simulink model "rlVarth_siml"  (R2020b)
settings: Solver=ode23t  StartTime=0.0  StopTime=Tf  RelTol=1e-2
model workspace: external: MAT-File C:\PhD\Variable Threshold\demo_rl.mat (data not in the file)
values from neighbouring files (symbols this model uses):
  A = [1.0000    0.1000;0    1.0000]    [RLenv.m]    (also in RlEnvModel.m; system.mat = [0.6278  -0.0259; 0.4644  0.7071]; systems_with_noise.m = [1.0000    0.1000; 0    1.0000])
  actorAtk = rlDeterministicActorRepresentation(actorNetwork,obsInfo{1,1},actInfo{1,1},'Observation',{'State'},'Action',{'Action'},actorOptions)    [demo_rl.m]    (also in main_rl.m = rlDeterministicActorRepresentation(actorNetwork,obsInfo{1,1}; main_rl_func_modified.m = rlDeterministicActorRepresentation(actorNetwork,obsInfo{1,1}; new_main_rl.m = rlDeterministicActorRepresentation(actorNetwork,obsInfo{1,1})
  actorCon = rlDeterministicActorRepresentation(actorNetwork,obsInfo{1,2},actInfo{1,2},'Observation',{'State'},'Action',{'Action'},actorOptions)    [demo_rl.m]    (also in main_rl.m = rlDeterministicActorRepresentation(actorNetwork,obsInfo{1,2}; main_rl_func_modified.m = rlDeterministicActorRepresentation(actorNetwork,obsInfo{1,2}; new_main_rl.m = rlDeterministicActorRepresentation(actorNetwork,obsInfo{1,2})
  actorDtc = rlDeterministicActorRepresentation(actorNetwork,obsInfo{1,3},actInfo{1,3},'Observation',{'State'},'Action',{'Action'},actorOptions)    [demo_rl.m]    (also in main_rl.m = rlDeterministicActorRepresentation(actorNetwork,obsInfo{1,3}; main_rl_func_modified.m = rlDeterministicActorRepresentation(actorNetwork,obsInfo{1,3}; new_main_rl.m = rlDeterministicActorRepresentation(actorNetwork,obsInfo{1,3})
  actuatorRange = [36]    [RLenv.m]    (also in RlEnvModel.m; system.mat = [0.8125 10000])
  agentOpts = rlDDPGAgentOptions(     'SampleTime',Ts,     'TargetSmoothFactor',1e-3,     'DiscountFactor',1.0,      'MiniBatchSize',64,      'ExperienceBufferLength',1e6)    [demo_rl.m]    (also in main_rl.m = rlDDPGAgentOptions(     'SampleTime',Ts,     'TargetSmoothFa; main_rl_func_modified.m = rlDDPGAgentOptions(     'SampleTime',Ts,     'TargetSmoothFa; new_main_rl.m = rlDDPGAgentOptions(     'SampleTime',Ts,     'TargetSmoothFa)
  B = [0.0050;0.1000]    [RLenv.m]    (also in RlEnvModel.m; system.mat = [0.1246  -2.8e-07; 3.2763  1.6e-05]; systems_with_noise.m = [0.0050; 0.1000])
  C = [1 0]    [RLenv.m]    (also in RlEnvModel.m; system.mat = [0  1; -338.7813  1.1293]; systems_with_noise.m)
  criticAtk = rlQValueRepresentation(criticNetwork,obsInfo{1,1},actInfo{1,1},'Observation',{'State'},'Action',{'Action'},criticOpts)    [demo_rl.m]    (also in main_rl.m = rlQValueRepresentation(criticNetwork,obsInfo{1,1},actInfo{1,; main_rl_func_modified.m = rlQValueRepresentation(criticNetwork,obsInfo{1,1},actInfo{1,; new_main_rl.m = rlQValueRepresentation(criticNetwork,obsInfo{1,1},actInfo{1,)
  criticCon = rlQValueRepresentation(criticNetwork,obsInfo{1,2},actInfo{1,2},'Observation',{'State'},'Action',{'Action'},criticOpts)    [demo_rl.m]    (also in main_rl.m = rlQValueRepresentation(criticNetwork,obsInfo{1,2},actInfo{1,; main_rl_func_modified.m = rlQValueRepresentation(criticNetwork,obsInfo{1,2},actInfo{1,; new_main_rl.m = rlQValueRepresentation(criticNetwork,obsInfo{1,2},actInfo{1,)
  criticDtc = rlQValueRepresentation(criticNetwork,obsInfo{1,3},actInfo{1,3},'Observation',{'State'},'Action',{'Action'},criticOpts)    [demo_rl.m]    (also in main_rl.m = rlQValueRepresentation(criticNetwork,obsInfo{1,3},actInfo{1,; main_rl_func_modified.m = rlQValueRepresentation(criticNetwork,obsInfo{1,3},actInfo{1,; new_main_rl.m = rlQValueRepresentation(criticNetwork,obsInfo{1,3},actInfo{1,)
  D = [0]    [RLenv.m]    (also in RlEnvModel.m; system.mat = [0  0; 169.3907  0]; systems_with_noise.m)
  K = [16.0302    5.6622]    [RLenv.m]    (also in RlEnvModel.m; system.mat = [5.261  -0.023; -414911.26  57009.48]; systems_with_noise.m)
  L = [0.9902;0.9892]    [RLenv.m]    (also in RlEnvModel.m; system.mat = [-2.708e-11  -6.3612e-10; 3.3671e-10  5.56308e-09]; systems_with_noise.m = [0.9902; 0.9892])
  sensorRange = [30000]    [RLenv.m]    (also in RlEnvModel.m; system.mat = [2.5 15])
  Ts = 0.1    [RLenv.m]    (also in RlEnvModel.m; demo_rl.m; main_rl.m = s.Ts; main_rl_func_modified.m = s.Ts)
undefined symbols (not defined in the file or in its folder): esp_env, rlDDPGAgent
libraries: rllib x3, simulink x2
settings Model: Creator=The MathWorks, Inc.  LastModifiedBy=IIT_KGP_CSE_FM_LAB

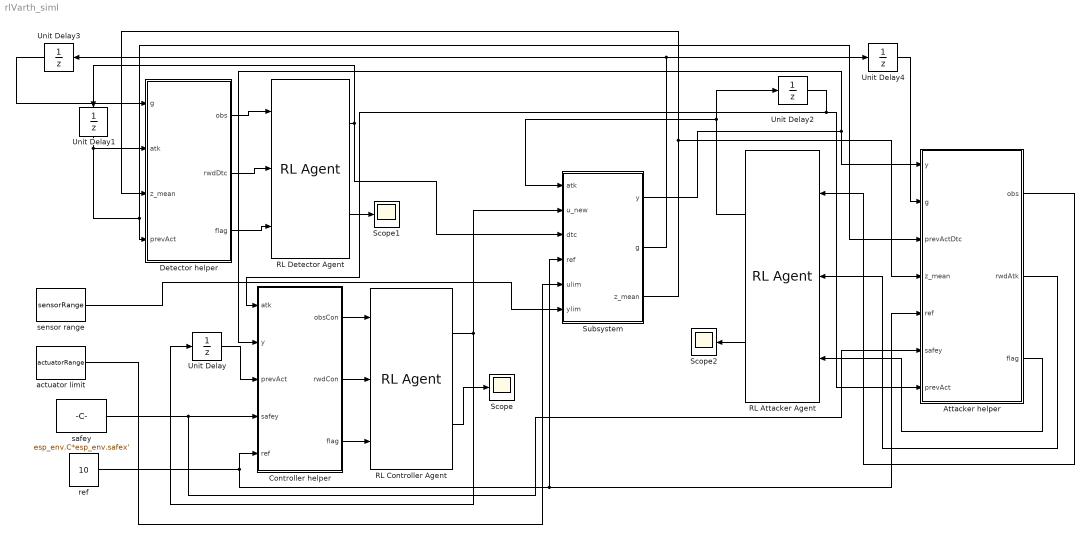
== system rlVarth_siml ==
  Attacker helper : Subsystem
  Controller helper : Subsystem
  Detector helper : Subsystem
  RL Attacker Agent : rllib/RL Agent  Agent=rlDDPGAgent(actorAtk,criticAtk,agentOpts)  ProvideReward=on  ProvideIsDone=on  ProvideCumRwd=on  TreatAsDirectFeedthrough=on  CollectLoggedSignals=on  CollectModelStates=on
  RL Controller Agent : rllib/RL Agent  Agent=rlDDPGAgent(actorCon,criticCon,agentOpts)  ProvideReward=on  ProvideIsDone=on  ProvideCumRwd=on  TreatAsDirectFeedthrough=on  CollectLoggedSignals=on  CollectModelStates=on
  RL Detector Agent : rllib/RL Agent  Agent=rlDDPGAgent(actorDtc,criticDtc,agentOpts)  ProvideReward=on  ProvideIsDone=on  ProvideCumRwd=on  TreatAsDirectFeedthrough=on  CollectLoggedSignals=on  CollectModelStates=on
  Scope : Scope
  Scope1 : Scope
  Scope2 : Scope
  Subsystem : Subsystem
  Unit Delay{,1..4} (5 alike) : UnitDelay  SampleTime=-1  HasFrameUpgradeWarning=on
  actuator limit : Constant  Value=actuatorRange
  ref : Constant  Value=10
  safey : Constant  Value=esp_env.C*esp_env.safex'
  sensor range : Constant  Value=sensorRange
  wires:
  RL Attacker Agent/1 -> Subsystem/1(atk), Unit Delay2/1
  ref/1 -> Attacker helper/5(ref), Subsystem/4(ref), Controller helper/5(ref)
  RL Controller Agent/1 -> Subsystem/2(u_new), Unit Delay/1
  RL Detector Agent/1 -> Subsystem/3(dtc), Unit Delay1/1
  RL Controller Agent/2 -> Scope/1
  RL Detector Agent/2 -> Scope1/1
  RL Attacker Agent/2 -> Scope2/1
  Unit Delay1/1 -> Attacker helper/3(prevActDtc), Detector helper/4(prevAct), Detector helper/2(atk)
  safey/1 -> Attacker helper/6(safey), Controller helper/4(safey)
  Subsystem/1(y) -> Attacker helper/1(y), Controller helper/2(y)
  Subsystem/2(g) -> Unit Delay4/1, Unit Delay3/1
  Subsystem/3(z_mean) -> Attacker helper/4(z_mean), Detector helper/3(z_mean)
  Detector helper/1(obs) -> RL Detector Agent/1
  Detector helper/2(rwdDtc) -> RL Detector Agent/2
  Detector helper/3(flag) -> RL Detector Agent/3
  Unit Delay2/1 -> Attacker helper/7(prevAct), Controller helper/1(atk)
  Unit Delay/1 -> Controller helper/3(prevAct)
  Controller helper/1(obsCon) -> RL Controller Agent/1
  Controller helper/2(rwdCon) -> RL Controller Agent/2
  Controller helper/3(flag) -> RL Controller Agent/3
  Attacker helper/1(obs) -> RL Attacker Agent/1
  Attacker helper/2(rwdAtk) -> RL Attacker Agent/2
  Attacker helper/3(flag) -> RL Attacker Agent/3
  Unit Delay3/1 -> Detector helper/1(g)
  Unit Delay4/1 -> Attacker helper/2(g)
  sensor range/1 -> Subsystem/6(ylim)
  actuator limit/1 -> Subsystem/5(ulim)

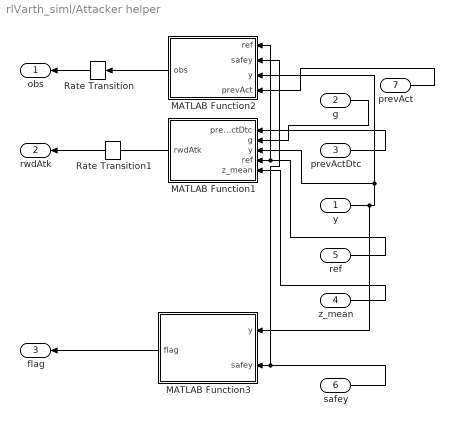
== system rlVarth_siml/Attacker helper ==
  y : Inport
  g : Inport  Port=2
  prevActDtc : Inport  Port=3
  z_mean : Inport  Port=4
  ref : Inport  Port=5
  safey : Inport  Port=6
  prevAct : Inport  Port=7
  MATLAB Function1 : MATLAB Function  TreatAsAtomicUnit=on
  MATLAB Function2 : MATLAB Function  TreatAsAtomicUnit=on
  MATLAB Function3 : MATLAB Function  TreatAsAtomicUnit=on
  Rate Transition : RateTransition
  Rate Transition1 : RateTransition
  obs : Outport
  rwdAtk : Outport  Port=2
  flag : Outport  Port=3
  wires:
  y/1 -> MATLAB Function2/3(y), MATLAB Function1/3(y), MATLAB Function3/1(y)
  g/1 -> MATLAB Function1/2(g)
  ref/1 -> MATLAB Function2/1(ref), MATLAB Function1/4(ref)
  MATLAB Function1/1(rwdAtk) -> rwdAtk/1
  z_mean/1 -> MATLAB Function1/5(z_mean)
  MATLAB Function3/1(flag) -> flag/1
  MATLAB Function2/1(obs) -> Rate Transition/1
  prevActDtc/1 -> MATLAB Function1/1(prevActDtc)
  safey/1 -> MATLAB Function2/2(safey), MATLAB Function3/2(safey)
  prevAct/1 -> MATLAB Function2/4(prevAct)
  Rate Transition/1 -> obs/1

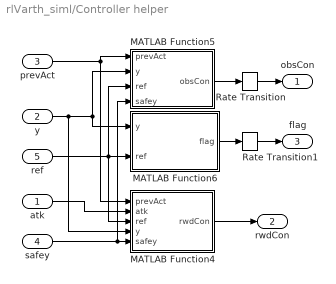
== system rlVarth_siml/Controller helper ==
  atk : Inport
  y : Inport  Port=2
  prevAct : Inport  Port=3
  safey : Inport  Port=4
  ref : Inport  Port=5
  MATLAB Function4 : MATLAB Function  TreatAsAtomicUnit=on
  MATLAB Function5 : MATLAB Function  TreatAsAtomicUnit=on
  MATLAB Function6 : MATLAB Function  TreatAsAtomicUnit=on
  Rate Transition : RateTransition
  Rate Transition1 : RateTransition
  obsCon : Outport
  rwdCon : Outport  Port=2
  flag : Outport  Port=3
  wires:
  ref/1 -> MATLAB Function4/3(ref), MATLAB Function6/2(ref), MATLAB Function5/3(ref)
  safey/1 -> MATLAB Function5/4(safey), MATLAB Function4/5(safey)
  MATLAB Function6/1(flag) -> Rate Transition1/1
  MATLAB Function4/1(rwdCon) -> rwdCon/1
  MATLAB Function5/1(obsCon) -> Rate Transition/1
  y/1 -> MATLAB Function6/1(y), MATLAB Function5/2(y), MATLAB Function4/4(y)
  prevAct/1 -> MATLAB Function4/1(prevAct), MATLAB Function5/1(prevAct)
  atk/1 -> MATLAB Function4/2(atk)
  Rate Transition/1 -> obsCon/1
  Rate Transition1/1 -> flag/1

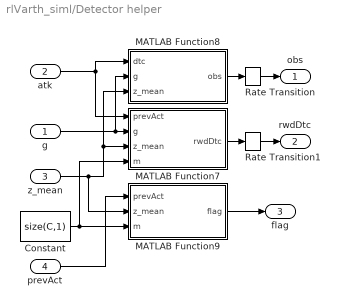
== system rlVarth_siml/Detector helper ==
  g : Inport
  atk : Inport  Port=2
  z_mean : Inport  Port=3
  prevAct : Inport  Port=4
  Constant : Constant  Value=size(C,1)  SampleTime=Ts
  MATLAB Function7 : MATLAB Function  TreatAsAtomicUnit=on
  MATLAB Function8 : MATLAB Function  TreatAsAtomicUnit=on
  MATLAB Function9 : MATLAB Function  TreatAsAtomicUnit=on
  Rate Transition : RateTransition  OutPortSampleTime=Ts
  Rate Transition1 : RateTransition
  obs : Outport
  rwdDtc : Outport  Port=2
  flag : Outport  Port=3
  wires:
  atk/1 -> MATLAB Function8/1(dtc), MATLAB Function7/1(prevAct)
  Constant/1 -> MATLAB Function9/3(m), MATLAB Function7/4(m)
  prevAct/1 -> MATLAB Function9/1(prevAct)
  z_mean/1 -> MATLAB Function9/2(z_mean), MATLAB Function7/3(z_mean), MATLAB Function8/3(z_mean)
  MATLAB Function8/1(obs) -> Rate Transition/1
  MATLAB Function7/1(rwdDtc) -> Rate Transition1/1
  g/1 -> MATLAB Function8/2(g), MATLAB Function7/2(g)
  MATLAB Function9/1(flag) -> flag/1
  Rate Transition/1 -> obs/1
  Rate Transition1/1 -> rwdDtc/1

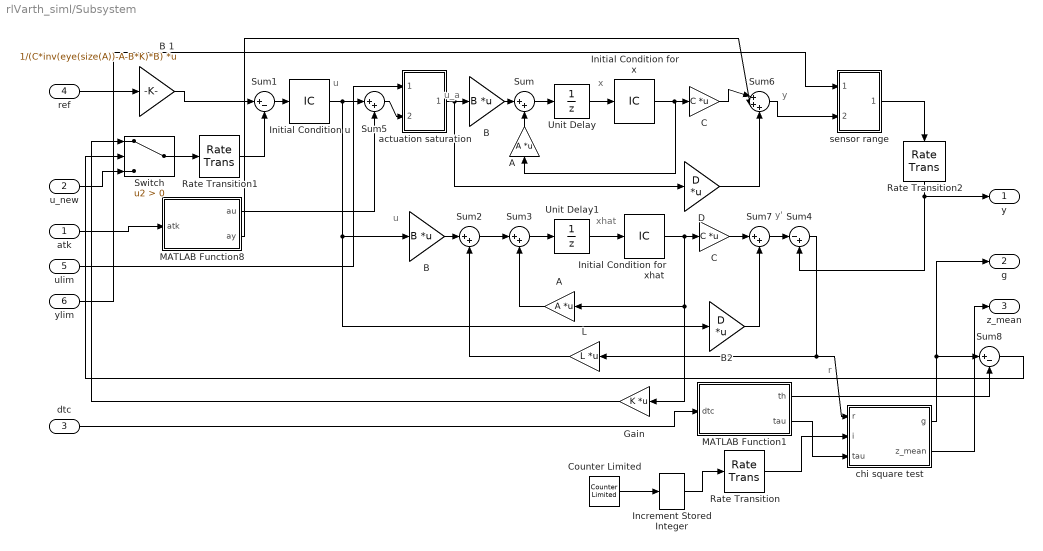
== system rlVarth_siml/Subsystem ==
  note: y
  note: r
  note: y'
  note: u
  note: u
  note: x
  note: xhat
  note: u_a
  atk : Inport
  u_new : Inport  Port=2
  dtc : Inport  Port=3
  ref : Inport  Port=4
  ulim : Inport  Port=5
  ylim : Inport  Port=6
  A : Gain  Gain=A  Multiplication=Matrix(K*u)
  "A " : Gain  Gain=A  Multiplication=Matrix(K*u)
  B : Gain  Gain=B  Multiplication=Matrix(K*u)
  "B " : Gain  Gain=B  Multiplication=Matrix(K*u)
  B 1 : Gain  Gain=1/(C*inv(eye(size(A))-A-B*K)*B)  Multiplication=Matrix(K*u)
  B2 : Gain  Gain=D  Multiplication=Matrix(K*u)
  C : Gain  Gain=C  Multiplication=Matrix(K*u)
  "C " : Gain  Gain=C  Multiplication=Matrix(K*u)
  Counter Limited : simulink/Sources/Counter Limited  uplimit=1/Ts-1  tsamp=Ts
  D : Gain  Gain=D  Multiplication=Matrix(K*u)
  Gain : Gain  Gain=K  Multiplication=Matrix(K*u)
  Increment Stored Integer : simulink/Additional Math & Discrete/Additional Math: Increment - Decrement/Increment Stored Integer
  Initial Condition u : InitialCondition  Value=zeros(size(B,2),1)
  Initial Condition for x : InitialCondition  Value=[0;0]
  Initial Condition for xhat : InitialCondition  Value=[0;0]
  L : Gain  Gain=L  Multiplication=Matrix(K*u)
  MATLAB Function1 : MATLAB Function  TreatAsAtomicUnit=on
  MATLAB Function8 : MATLAB Function  TreatAsAtomicUnit=on
  Rate Transition : RateTransition  OutPortSampleTime=Ts
  Rate Transition1 : RateTransition  OutPortSampleTime=Ts
  Rate Transition2 : RateTransition  OutPortSampleTime=Ts
  Sum{,2..3,5,7} (5 alike) : Sum  Inputs=|++
  Sum1 : Sum  Inputs=|+-
  Sum4 : Sum  Inputs=|-+
  Sum6 : Sum  Inputs=|+++
  Sum8 : Sum  Inputs=|+-
  Switch : Switch  Criteria=u2 > Threshold
  Unit Delay : UnitDelay  SampleTime=-1  HasFrameUpgradeWarning=on
  Unit Delay1 : UnitDelay  SampleTime=-1  HasFrameUpgradeWarning=on
  actuation saturation : Subsystem
  chi square test : Subsystem
  sensor range : Subsystem
  y : Outport
  g : Outport  Port=2
  z_mean : Outport  Port=3
  wires:
  Initial Condition for xhat/1 -> C/1, A/1, Gain/1
  L/1 -> Sum2/2
  "C "/1 -> Sum6/1
  D/1 -> Sum6/3
  u_new/1 -> Switch/3
  Unit Delay1/1 -> Initial Condition for xhat/1
  Sum7/1 -> Sum4/1
  Sum4/1 -> chi square test/1(r), L/1
  Sum3/1 -> Unit Delay1/1
  Unit Delay/1 -> Initial Condition for x/1
  Sum2/1 -> Sum3/1
  Sum1/1 -> Initial Condition u/1
  Initial Condition u/1 -> B/1, B2/1, Sum5/1
  Gain/1 -> Switch/1
  B2/1 -> Sum7/2
  actuation saturation/1(Out1) -> D/1, "B "/1
  A/1 -> Sum3/2
  Sum5/1 -> actuation saturation/2(In3)
  "B "/1 -> Sum/1
  Sum6/1 -> sensor range/2(In3)
  C/1 -> Sum7/1
  "A "/1 -> Sum/2
  Initial Condition for x/1 -> "C "/1, "A "/1
  ref/1 -> B 1/1
  B/1 -> Sum2/1
  Switch/1 -> Rate Transition1/1
  Sum/1 -> Unit Delay/1
  Sum8/1 -> Switch/2
  atk/1 -> MATLAB Function8/1(atk)
  MATLAB Function8/1(au) -> Sum5/2
  MATLAB Function8/2(ay) -> Sum6/2
  B 1/1 -> Sum1/1
  dtc/1 -> MATLAB Function1/1(dtc)
  MATLAB Function1/2(tau) -> chi square test/3(tau)
  chi square test/1(g) -> g/1, Sum8/1
  MATLAB Function1/1(th) -> Sum8/2
  ulim/1 -> actuation saturation/1(lim)
  sensor range/1(y_obs) -> Rate Transition2/1
  ylim/1 -> sensor range/1(lim)
  chi square test/2(z_mean) -> z_mean/1
  Increment Stored Integer/1 -> Rate Transition/1
  Counter Limited/1 -> Increment Stored Integer/1
  Rate Transition/1 -> chi square test/2(i)
  Rate Transition1/1 -> Sum1/2
  Rate Transition2/1 -> y/1, Sum4/2

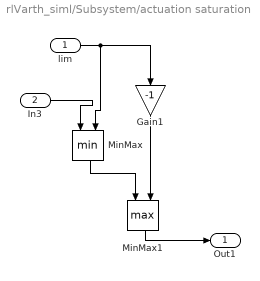
== system rlVarth_siml/Subsystem/actuation saturation ==
  lim : Inport
  In3 : Inport  Port=2
  Gain1 : Gain  Gain=-1
  MinMax : MinMax  Inputs=2
  MinMax1 : MinMax  Function=max  Inputs=2
  Out1 : Outport
  wires:
  Gain1/1 -> MinMax1/2
  MinMax/1 -> MinMax1/1
  MinMax1/1 -> Out1/1
  lim/1 -> Gain1/1, MinMax/2
  In3/1 -> MinMax/1

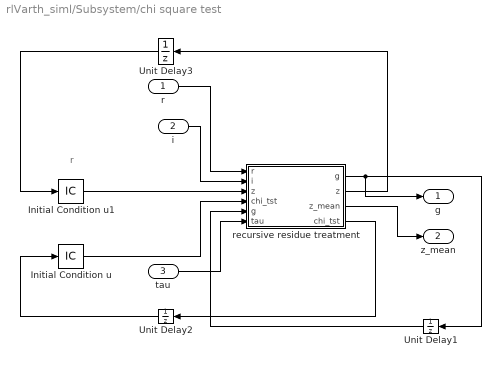
== system rlVarth_siml/Subsystem/chi square test ==
  note: r
  r : Inport
  i : Inport  Port=2
  tau : Inport  Port=3
  Initial Condition u : InitialCondition  Value=[0]
  Initial Condition u1 : InitialCondition  Value=[0]
  Unit Delay1 : UnitDelay  SampleTime=Ts  HasFrameUpgradeWarning=on
  Unit Delay2 : UnitDelay  SampleTime=Ts  HasFrameUpgradeWarning=on
  Unit Delay3 : UnitDelay  InitialCondition=[0]  SampleTime=Ts  HasFrameUpgradeWarning=on
  recursive residue treatment : MATLAB Function  TreatAsAtomicUnit=on
  g : Outport
  z_mean : Outport  Port=2
  wires:
  Unit Delay2/1 -> Initial Condition u/1
  Initial Condition u1/1 -> recursive residue treatment/3("z ")
  r/1 -> recursive residue treatment/1(r)
  Unit Delay1/1 -> recursive residue treatment/5("g ")
  Initial Condition u/1 -> recursive residue treatment/4("chi_tst ")
  Unit Delay3/1 -> Initial Condition u1/1
  recursive residue treatment/3(z_mean) -> z_mean/1
  i/1 -> recursive residue treatment/2(i)
  recursive residue treatment/4(chi_tst) -> Unit Delay2/1
  tau/1 -> recursive residue treatment/6(tau)
  recursive residue treatment/2(z) -> Unit Delay3/1
  recursive residue treatment/1(g) -> Unit Delay1/1, g/1

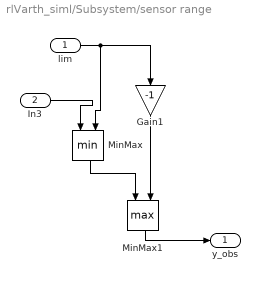
== system rlVarth_siml/Subsystem/sensor range ==
  lim : Inport
  In3 : Inport  Port=2
  Gain1 : Gain  Gain=-1
  MinMax : MinMax  Inputs=2
  MinMax1 : MinMax  Function=max  Inputs=2
  y_obs : Outport
  wires:
  Gain1/1 -> MinMax1/2
  MinMax/1 -> MinMax1/1
  MinMax1/1 -> y_obs/1
  lim/1 -> Gain1/1, MinMax/2
  In3/1 -> MinMax/1

== matlab function rlVarth_siml/Detector helper/MATLAB Function9 ==
  data: prevAct input; flag output; z_mean input; m input
function flag  = stopDtc(prevAct,z_mean,m)
   th= prevAct(1);
   tau = prevAct(2,1);
   dof = m*(tau);
   FAR = 1-chi2cdf(th,dof);
   TPR = 1- ncx2cdf(th,dof,z_mean)
   flag=0;
   if FAR < 0.004 & TPR > 0.96
       flag=1;
   end

== matlab function rlVarth_siml/Subsystem/MATLAB Function8 ==
  data: au output; atk input; ay output
function [au,ay] = atkParams(atk)
    au= atk(1);
    ay= atk(2);

== matlab function rlVarth_siml/Subsystem/chi square test/recursive residue treatment ==
  data: g output; r input; i input; z input; z output; z_mean output; chi_tst output; chi_tst input; g input; tau input
function [g,z,z_mean,chi_tst] = fcn(r,i,z,chi_tst,g,tau)
i
z(i)=r
z_mean=mean(z)
P= size(z',1)
chi_tst(i)= z(:,i)'*z(:,i)/P
g(i) = 0;              
for k = max(1,i-tau+1):i
    g(i) = g(i) + chi_tst(k)  % Calculate gk (chi2 test)
end

== matlab function rlVarth_siml/Attacker helper/MATLAB Function1 ==
  data: rwdAtk output; prevActDtc input; g input; y input; ref input; z_mean input
function rwdAtk  = rwrdAtk(prevActDtc,g,y,ref,z_mean)
   th= prevActDtc(1);
   tau = prevActDtc(2,1);
   dof = size(y,1)*(tau);
   FAR = 1-chi2cdf(th,dof);
   TPR = 1- ncx2cdf(th,dof,z_mean)
   rwdAtk = FAR/TPR + 50*(g<th)+ 100*(y-ref)^2;

== matlab function rlVarth_siml/Subsystem/MATLAB Function1 ==
  data: th output; dtc input; tau output
function [th,tau] = dtcParams(dtc)
    th= dtc(1);
    tau= dtc(2);

== matlab function rlVarth_siml/Attacker helper/MATLAB Function2 ==
  data: obs output; ref input; safey input; y input; prevAct input
function obs = obsAtk(ref,safey,y,prevAct)
    obs= [ref;y;safey;prevAct];

== matlab function rlVarth_siml/Attacker helper/MATLAB Function3 ==
  data: y input; flag output; safey input
function flag  = stop(y,safey)
    flag = y >safey;

== matlab function rlVarth_siml/Controller helper/MATLAB Function4 ==
  data: rwdCon output; prevAct input; atk input; ref input; y input; safey input
function rwdCon  = rwrdCon(prevAct,atk,ref,y,safey)
    au=atk(1);
    ay=atk(2);
    rwdCon = -(prevAct+au)^2-20*(y-ref)^2-200*(abs(y) > safey);

== matlab function rlVarth_siml/Controller helper/MATLAB Function5 ==
  data: obsCon output; prevAct input; y input; ref input; safey input
function obsCon = obsCon(prevAct,y,ref,safey)
   
    obsCon=[prevAct;y;ref;safey];

== matlab function rlVarth_siml/Controller helper/MATLAB Function6 ==
  data: y input; ref input; flag output
function flag  = stop(y,ref)
    
    flag= abs(y-ref) == 0;

== matlab function rlVarth_siml/Detector helper/MATLAB Function7 ==
  data: rwdDtc output; prevAct input; g input; z_mean input; m input
function rwdDtc  = rwrdDtc(prevAct,g,z_mean,m)
   th= prevAct(1);
   tau = prevAct(2,1);
   dof = m*(tau);
   FAR = 1-chi2cdf(th,dof);
   TPR = 1- ncx2cdf(th,dof,z_mean)
   rwdDtc = TPR/FAR + 50*(g<=th);

== matlab function rlVarth_siml/Detector helper/MATLAB Function8 ==
  data: obs output; dtc input; g input; z_mean input
function obs = obsDtc(dtc,g,z_mean)
    obs=[dtc;g(end);z_mean];
